simulink model "CNblk"  (Simulink 6.5)
settings: Solver=ode45  SolverMode=SingleTasking  StartTime=0.0  StopTime=999999  MaxStep=10  RelTol=1e-3  AbsTol=1e-3
undefined symbols (not defined in the file): k, TI
settings Model: Creator=lfd  LastModifiedBy=lfd  ExtModeAutoUpdateStatusClock=off
settings DataIOCC: LimitDataPoints=off  SaveOutput=off  SaveTime=off
settings OptimizationCC: BlockReduction=off  BooleanDataType=off
settings DebuggingCC: SolverPrmCheckMsg=none  MultiTaskDSMMsg=warning  MultiTaskCondExecSysMsg=none  StrictBusMsg=None
settings HardwareCC: TargetUnknown=on
settings RTWCC: IncludeERTFirstTime=on
settings GRTTargetCC: ModelReferenceCompliant=off  MatFileLogging=off

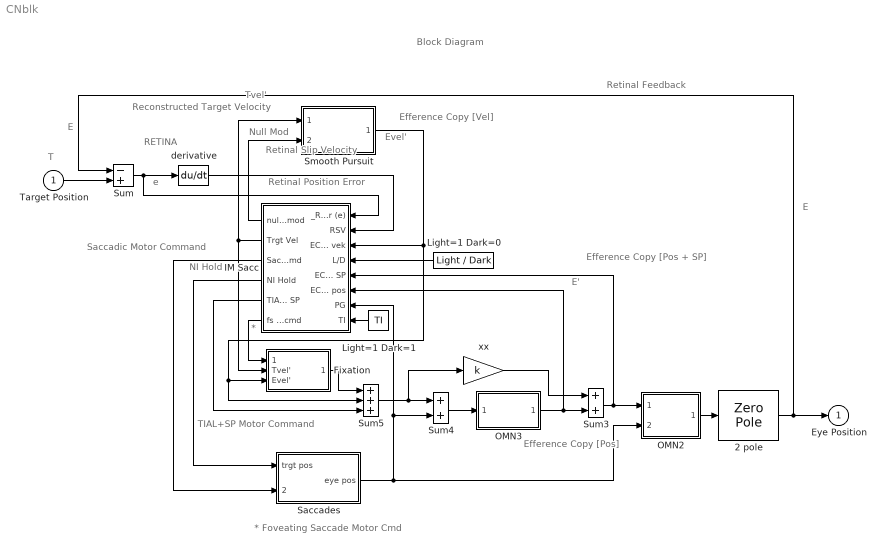
== system CNblk ==
  note: Block Diagram
  note: TIAL+SP
      | Motor Command
  note: NI Hold
  note: Saccadic Motor
      | Command
  note: Efference Copy
      | [Vel]
  note: Reconstructed
      | Target Velocity
  note: Efference Copy
      | [Pos]
  note: Efference Copy
      | [Pos + SP]
  note: Retinal Position Error
  note: E
  note: e
  note: E
  note: T
  note: Retinal Feedback
  note: Evel'
  note: E'
  note: Tvel'
  note: Retinal Slip Velocity
  note: RETINA
  note: *
  note: * Foveating Saccade Motor Cmd
  note: Null Mod
  Target Position : Inport
  2 pole : ZeroPole  Zeros=[ ]  Poles=[ -1/.18 -1/.007]  Gain=[1/.18 * 1/.007]
      mask Display: disp('EOM\n[2-Pole\nPlant]')
  Fixation : Subsystem
      mask Display: disp('Fixation')
  IM Sacc : Subsystem  Orientation=left
      mask Display: disp('INTERNAL\nMONITOR\n[Sacc,FS/BS,\nSP,AL,\nNI Control]')
  Light=1 Dark=0 : Constant  Orientation=left  Value=Light / Dark
  Light=1 Dark=1 : Constant  Orientation=left  Value=TI
  OMN2 : Subsystem
      mask Display: disp('OMN\n[Tonic +\nPhasic]')
  OMN3 : Subsystem
      mask Display: disp('Neural \nIntegrator')
  Saccades : Subsystem
      mask Display: disp('Saccadic\n[PG,NI Hold]')
  Smooth Pursuit : Subsystem
      mask Display: disp('Smooth\nPursuit')
  Sum : Sum  Inputs=-+  SaturateOnIntegerOverflow=on  InputSameDT=on
  Sum3 : Sum  SaturateOnIntegerOverflow=on  InputSameDT=on
  Sum4 : Sum  SaturateOnIntegerOverflow=on  InputSameDT=on
  Sum5 : Sum  Inputs=+++  SaturateOnIntegerOverflow=on  InputSameDT=on
  derivative : Derivative
      mask Display: disp('s')
  xx : Gain  Gain=k  SaturateOnIntegerOverflow=on
  Eye Position : Outport  InitialOutput=0
  wires:
  derivative/1 -> IM Sacc/2(RSV)
  Sum/1 -> IM Sacc/1(_RetErr (e)), derivative/1
  Target Position/1 -> Sum/2
  Light=1 Dark=0/1 -> IM Sacc/4(L/D)
  xx/1 -> Sum3/1
  Saccades/1(eye pos) -> Sum4/2, IM Sacc/7(PG), OMN2/2(from PG)
  Light=1 Dark=1/1 -> IM Sacc/8(TI)
  OMN3/1(out_1) -> IM Sacc/6(ECPY pos), Sum3/2
  Sum3/1 -> IM Sacc/5(ECPY P + SP), OMN2/1(from NI)
  OMN2/1(out_1) -> 2 pole/1
  2 pole/1 -> Eye Position/1, Sum/1
  Sum4/1 -> OMN3/1(from NI)
  Smooth Pursuit/1(eye pos) -> IM Sacc/3(ECPY vek), Fixation/3(Evel'), Sum5/2
  Fixation/1(" CorrVel [velcorr]") -> Sum5/1
  Sum5/1 -> Sum4/1, xx/1
  IM Sacc/6(fs mot cmd) -> Fixation/1(fs [fsmc30])
  IM Sacc/1(null mod) -> Smooth Pursuit/2(null mod)
  IM Sacc/5(TIAL + SP) -> Sum5/3
  IM Sacc/4(NI Hold) -> Saccades/1(trgt pos)
  IM Sacc/3(Sacc Mot Cmd) -> Saccades/2()
  IM Sacc/2(Trgt Vel) -> Smooth Pursuit/1(trgt pos), Fixation/2(Tvel')

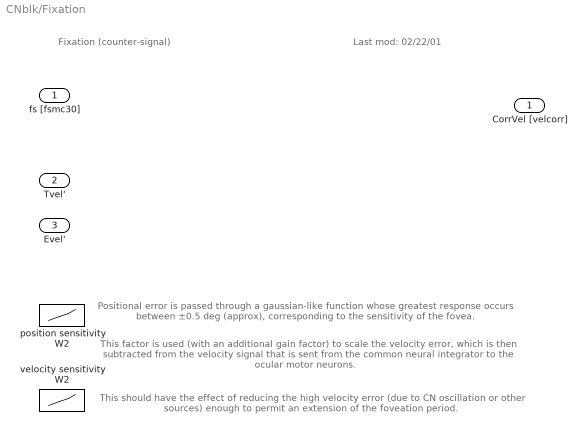
== system CNblk/Fixation ==
  note: Fixation (counter-signal)
  note: Last mod: 02/22/01
  note: Positional error is passed through a gaussian-like function whose greatest
      | response occurs between ±0.5 deg (approx), corresponding to the sensitivity
      | of the fovea.
  note: This factor is used (with an additional gain factor) to scale the velocity error,
      | which is then subtracted from the velocity signal that is sent from the
      | common neural integrator to the ocular motor neurons.
  note: This should have the effect of reducing the high velocity error (due
      | to CN oscillation or other sources) enough to permit an extension of
      | the foveation period.
  fs [fsmc30] : Inport
  Tvel' : Inport  Port=2
  Evel' : Inport  Port=3
  position sensitivity W2 : Lookup  InputValues="[-5 -2  -1 -0.5   0.5   1    2    5]"  OutputValues="[ 0   0.125    0.5     1      1     0.5    0.125  0]"  SaturateOnIntegerOverflow=on
  velocity sensitivity W2 : Lookup  InputValues="[-30 -15   -8  -4   4     8  15  30]"  OutputValues="[0  0.125   0.5    1    1    0.5   0.125  0]"  SaturateOnIntegerOverflow=on
  " CorrVel [velcorr]" : Outport  InitialOutput=0
  wires:
  ? -> " CorrVel [velcorr]"/1

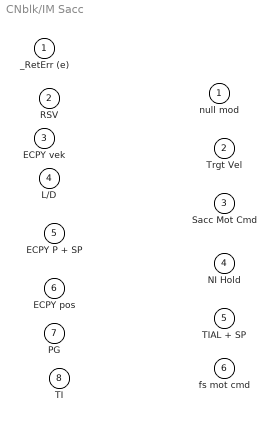
== system CNblk/IM Sacc ==
  _RetErr (e) : Inport
  RSV : Inport  Port=2
  ECPY vek : Inport  Port=3
  L/D : Inport  Port=4
  ECPY P + SP : Inport  Port=5
  ECPY pos : Inport  Port=6
  PG : Inport  Port=7
  TI : Inport  Port=8
  null mod : Outport  InitialOutput=0
  Trgt Vel : Outport  Port=2  InitialOutput=0
  Sacc Mot Cmd : Outport  Port=3  InitialOutput=0
  NI Hold : Outport  Port=4  InitialOutput=0
  TIAL + SP : Outport  Port=5  InitialOutput=0
  fs mot cmd : Outport  Port=6  InitialOutput=0

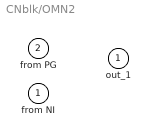
== system CNblk/OMN2 ==
  from NI : Inport
  from PG : Inport  Port=2
  out_1 : Outport  InitialOutput=0

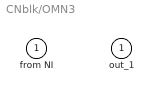
== system CNblk/OMN3 ==
  from NI : Inport
  out_1 : Outport  InitialOutput=0

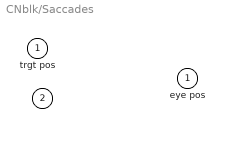
== system CNblk/Saccades ==
  trgt pos : Inport
   : Inport  Port=2
  eye pos : Outport  InitialOutput=0

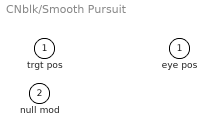
== system CNblk/Smooth Pursuit ==
  trgt pos : Inport
  null mod : Inport  Port=2
  eye pos : Outport  InitialOutput=0
